simulink model "RmRmRmUS_Simulink"  (R2015a)
settings: Solver=ode3  StartTime=0.0  StopTime=tf  FixedStep=t_step  RelTol=1e-3
values from neighbouring files (symbols this model uses):
  a0 = theta0    (= 0)    [Kinematics.m]    (also in RmRmRmUS.m)
  a1 = dtheta0    (= 0)    [Kinematics.m]    (also in RmRmRmUS.m)
  a2 = ddtheta0/2    (= 0)    [Kinematics.m]    (also in RmRmRmUS.m)
  a3 = ( 20*(thetaf - theta0)        - (8*dthetaf + 12*dtheta0)*tf        - (3*ddtheta0 - ddthetaf)*tf^2 ) / (2*tf^3)    [Kinematics.m]    (also in RmRmRmUS.m = ( 20*(thetaf - theta0)        - (8*dthetaf + 12*dtheta0)*tf_)
  a4 = ( -30*(thetaf - theta0)        + (14*dthetaf + 16*dtheta0)*tf        + (3*ddtheta0 - 2*ddthetaf)*tf^2 ) / (2*tf^4)    [Kinematics.m]    (also in RmRmRmUS.m = ( -30*(thetaf - theta0)        + (14*dthetaf + 16*dtheta0)*t)
  a5 = ( 12*(thetaf - theta0)        - (6*dthetaf + 6*dtheta0)*tf        - (ddtheta0 - ddthetaf)*tf^2 ) / (2*tf^5)    [Kinematics.m]    (also in RmRmRmUS.m = ( 12*(thetaf - theta0)        - (6*dthetaf + 6*dtheta0)*tf_i)
  dqI0 = [0; 0]    [RmRmRmUS.m]
  g = 9.8    [RmRmRmUS.m]
  J1 = 0.1    [RmRmRmUS.m]
  J2 = 0.1    [RmRmRmUS.m]
  J3 = 0.1    [RmRmRmUS.m]
  Kd = [1; 1; 1] * (8/t_stl)    [RmRmRmUS.m]
  Kp = [1; 1; 1] * (4/t_stl)^2    [RmRmRmUS.m]
  l1 = 0.2    [Kinematics.m]    (also in RmRmRmUS.m)
  l2 = 0.2    [Kinematics.m]    (also in RmRmRmUS.m)
  l3 = 1    [Kinematics.m]    (also in RmRmRmUS.m)
  l4 = 1    [Kinematics.m]    (also in RmRmRmUS.m)
  lB = 1    [Kinematics.m]    (also in RmRmRmUS.m)
  lG2 = l2/2    (= 0.1)    [RmRmRmUS.m]
  lG3 = l3/2    (= 0.5)    [RmRmRmUS.m]
  m2 = 1    [RmRmRmUS.m]
  m3 = 1    [RmRmRmUS.m]
  ndv = (qBf-qB0) / norm(qBf-qB0)    [Kinematics.m]    (also in RmRmRmUS.m = (qBf-qB0) / thetaf)
  qB0 = [deg2rad(185); deg2rad(10)]    [Kinematics.m]    (also in RmRmRmUS.m)
  qD0 = [q3_0; qB0]    [RmRmRmUS.m]
  qI0 = [q1_0; q2_0]    [RmRmRmUS.m]
  T0 = [0; 0; 0]    [RmRmRmUS.m]
  tf_ik = 1    [RmRmRmUS.m]
  x0S = 0    [Kinematics.m]    (also in RmRmRmUS.m)
  y0S = 2.5    [Kinematics.m]    (also in RmRmRmUS.m)
  z0S = 0.5    [Kinematics.m]    (also in RmRmRmUS.m)
settings Model: Creator=Marcelo  LastModifiedBy=Marcelo

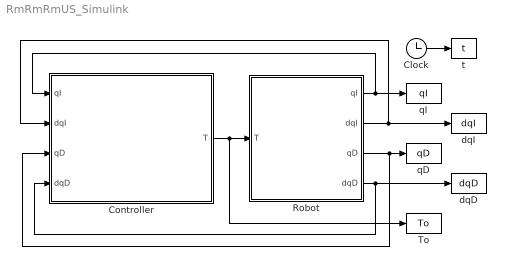
== system RmRmRmUS_Simulink ==
  Clock : Clock
  Controller : Subsystem
      mask Display: image(imread('Circuit.png'))
  Robot : Subsystem
      mask Display: image(imread('RobotPic.png'))
  To : ToWorkspace  VariableName=To  SampleTime=-1
  dqD : ToWorkspace  VariableName=dqD  SampleTime=-1
  dqI : ToWorkspace  VariableName=dqI  SampleTime=-1
  qD : ToWorkspace  VariableName=qD  SampleTime=-1
  qI : ToWorkspace  VariableName=qI  SampleTime=-1
  t : ToWorkspace  VariableName=t  SampleTime=-1
  wires:
  Robot/1(qI) -> qI/1, Controller/1(qI)
  Robot/3(qD) -> qD/1, Controller/3(qD)
  Robot/4(dqD) -> dqD/1, Controller/4(dqD)
  Robot/2(dqI) -> dqI/1, Controller/2(dqI)
  Clock/1 -> t/1
  Controller/1(T) -> To/1, Robot/1(T)

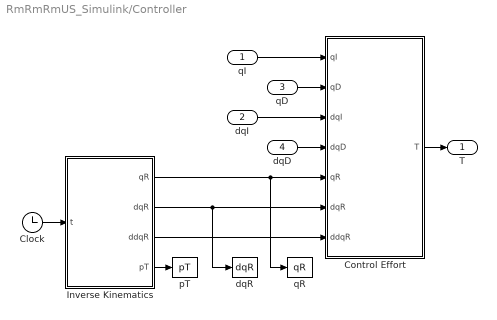
== system RmRmRmUS_Simulink/Controller ==
  qI : Inport
  dqI : Inport  Port=2
  qD : Inport  Port=3
  dqD : Inport  Port=4
  Clock : Clock
  Control Effort : MATLAB Function  TreatAsAtomicUnit=on
  Inverse Kinematics : MATLAB Function  TreatAsAtomicUnit=on
  dqR : ToWorkspace  VariableName=dqR  SampleTime=-1
  pT : ToWorkspace  VariableName=pT  SampleTime=-1
  qR : ToWorkspace  VariableName=qR  SampleTime=-1
  T : Outport
  wires:
  Inverse Kinematics/1(qR) -> qR/1, Control Effort/5(qR)
  Inverse Kinematics/2(dqR) -> dqR/1, Control Effort/6(dqR)
  Inverse Kinematics/3(ddqR) -> Control Effort/7(ddqR)
  Clock/1 -> Inverse Kinematics/1(t)
  dqD/1 -> Control Effort/4(dqD)
  dqI/1 -> Control Effort/3(dqI)
  qD/1 -> Control Effort/2(qD)
  qI/1 -> Control Effort/1(qI)
  Control Effort/1(T) -> T/1
  Inverse Kinematics/4(pT) -> pT/1

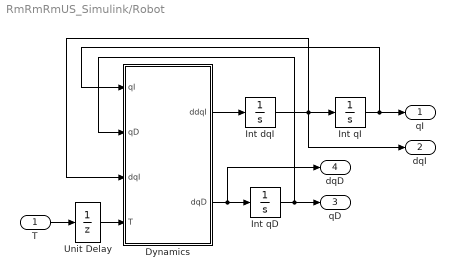
== system RmRmRmUS_Simulink/Robot ==
  T : Inport
  Dynamics : MATLAB Function  TreatAsAtomicUnit=on
  Int dqI : Integrator  InitialCondition=dqI0
  Int qD : Integrator  InitialCondition=qD0
  Int qI : Integrator  InitialCondition=qI0
  Unit Delay : UnitDelay  InitialCondition=T0  SampleTime=-1
  qI : Outport
  dqI : Outport  Port=2
  qD : Outport  Port=3
  dqD : Outport  Port=4
  wires:
  Dynamics/1(ddqI) -> Int dqI/1
  Int qI/1 -> qI/1, Dynamics/1(qI)
  Int dqI/1 -> Dynamics/3(dqI), dqI/1, Int qI/1
  Dynamics/2(dqD) -> dqD/1, Int qD/1
  T/1 -> Unit Delay/1
  Int qD/1 -> qD/1, Dynamics/2(qD)
  Unit Delay/1 -> Dynamics/4(T)

== matlab function RmRmRmUS_Simulink/Controller/Control Effort ==
  data: qI input; T output double; qD input; dqI input; dqD input; qR input; dqR input; ddqR input; Kp parameter; Kd parameter; lG2 parameter; l3 parameter; lG3 parameter; m2 parameter; m3 parameter; g parameter; J1 parameter; J2 parameter; J3 parameter
function T  = fcn(qI, qD, dqI, dqD, qR, dqR, ddqR, Kp, Kd, lG2, l3, ...
    lG3, m2, m3, g, J1, J2, J3)
%%% FEEDBACK LINEARIZATION
q = [qI; qD(1)];
dq = [dqI; dqD(1)];
v = ddqR - Kp.*(q-qR) - Kd.*(dq-dqR);
q2 = qI(2);
q3 = qD(1);
dq1 = dqI(1);
dq2 = dqI(2);
dq3 = dqD(1);
% RRR robotic arm dynamics
H = mtxH_RRR (q2, q3, dq1, dq2, dq3, lG2, l3, lG3, m2, m3);
G = vecG_RRR (q2, q3, lG2, l3, lG3, m2, m3, g);
M = mtxM_RRR (q2, q3, lG2, l3, lG3, J1, J2, J3, m2, m3);
T = H*dq + G + M*v;

== matlab function RmRmRmUS_Simulink/Robot/Dynamics ==
  data: qI input; qD input; dqI input; T input double; ddqI output; dqD output; l3 parameter; l4 parameter; lB parameter; lG2 parameter; lG3 parameter; J1 parameter; J2 parameter; J3 parameter; m2 parameter; m3 parameter; g parameter
function [ddqI, dqD] = fcn(qI, qD, dqI, T, l3, l4, lB, lG2, lG3, J1, ...
    J2, J3, m2, m3, g)

q1 = qI(1);
q2 = qI(2);

q3 = qD(1);
q4 = qD(2);
q5 = qD(3);

dq1 = dqI(1);
dq2 = dqI(2);

T1 = T(1);
T2 = T(2);
T3 = T(3);

dq3 = vg_dq3(q1, q2, q3, q4, q5, dq1, dq2, l3, l4);
dq4 = vg_dq4(q1, q2, q3, q4, q5, dq1, dq2, l3, l4, lB);
dq5 = vg_dq5(q1, q2, q3, q4, q5, dq1, dq2, l3, l4, lB);

M = mtxM(q1, q2, q3, q4, q5, lG2, l3, lG3, l4, J1, J2, J3, m2, m3);
H = mtxH(q1, q2, q3, q4, q5, dq1, dq2, dq3, dq4, dq5, lG2, l3, lG3, ...
    l4, J3, m2, m3);
G = vecG(q1, q2, q3, q4, q5, lG2, l3, lG3, l4, m2, m3, g);
To = vecT (q1, q2, q3, q4, q5, l3, l4, T1, T2, T3);

dqD = [dq3; dq4; dq5];
ddqI = M\(To - G - H*dqI);

== matlab function RmRmRmUS_Simulink/Controller/Inverse Kinematics ==
  data: t input; qR output; dqR output; ddqR output; pT output; qB0 parameter; tf_ik parameter; a0 parameter; a1 parameter; a2 parameter; a3 parameter; a4 parameter; a5 parameter; ndv parameter; lB parameter; x0S parameter; y0S parameter; z0S parameter; l1 parameter; l2 parameter; l3 parameter; l4 parameter
function [qR, dqR, ddqR, pT] = fcn(t, qB0, tf_ik, a0, a1, a2, a3, a4, ...
    a5, ndv, lB, x0S, y0S, z0S, l1, l2, l3, l4)
% Time limit
if t > tf_ik
    t = tf_ik;
end

%%% QUINTIC POLYNOMIAL
theta = a0 + a1*t + a2*t.^2 + a3*t.^3 + a4*t.^4 + a5*t.^5;
dtheta = a1 + 2*a2*t + 3*a3*t.^2 + 4*a4*t.^3 + 5*a5*t.^4;
ddtheta = 2*a2 + 6*a3*t + 12*a4*t.^2 + 20*a5*t.^3;
%%% CUBIC POLYNOMIAL
%theta = a0 + a1*t + a2*t^2 + a3*t^3;
%dtheta = a1 + 2*a2*t + 3*a3*t^2;
%ddtheta = 2*a2 + 6*a3*t;
% Bar generalized coordinates q4 and q5
qB = qB0 + theta * ndv; % Bar generalized coordinates
dqB = dtheta * ndv; % Bar generalized velocities
ddqB = ddtheta * ndv; % Bar generalized accelerations
% Bar generalized coordinates
q4 = qB(1);
q5 = qB(2);
% Bar generalized velocities
dq4 = dqB(1);
dq5 = dqB(2);

%%% BAR DIRECT KINEMATICS
% Tool position
pxT = - cos(q5) * sin(q4) * lB + x0S;
pyT = cos(q5) * cos(q4) * lB + y0S;
pzT = sin(q5) * lB + z0S;
pT = [pxT; pyT; pzT];
% Tool velocity and acceleration
JqB = mtx_JqB(q4, q5, lB);
dJqB = mtx_dJqB(q4, q5, dq4, dq5, lB);
vT = JqB * dqB;
aT = dJqB * dqB + JqB * ddqB;

%%% ROBOTIC ARM INVERSE KINEMATICS
dzT = pzT - l1 - l2;
Rxy = sqrt(pxT^2 + pyT^2);
% Robotic arm generalized coordinates
q1 = asin(-pxT/Rxy);
q3 = -acos((Rxy^2+dzT^2-l3^2-l4^2)/(2*l3*l4));
q2 = -asin(((l3+l4*cos(q3))*Rxy+l4*sin(q3)*dzT)/...
    (l3^2+2*l3*l4*cos(q3)+l4^2));
qR = [q1; q2; q3];
% Robotic arm generalized velocities and accelerations
if t > tf_ik % Time limit
    dqR = [0; 0; 0];
    ddqR = [0; 0; 0];
else
    iJqR = mtx_invJqR(q1, q2, q3, l3, l4);
    dqR = iJqR * vT;
    dJqR = mtx_dJqR(q1, q2, q3, dqR(1), dqR(2), dqR(3), l3, l4);
    ddqR = iJqR * (aT - dJqR * dqR);
end
